simulink model "ACStesbed1"  (R2013b)
settings: Solver=ode45  StartTime=0.0  StopTime=10000  FixedStep=0.01  RelTol=1e-3
StartFcn:
  | InitializeModel
undefined symbols (not defined in the file or in its folder): DiscIntNeverNeededParam, e0_0, e1_0, e2_0, e3_0, magnitude, OrbData, params
libraries: aerolibutil x29, vrlib x26, satellite_control_lib x17, aerolibtransform2 x5, dspmtrx3 x5, aerolib6dofsys x4, dspinverses x3, simulink x3, aerolib6dof2 x1
(part 1 of 2)
settings Model: Creator=DNikolaev  LastModifiedBy=DNikolaev

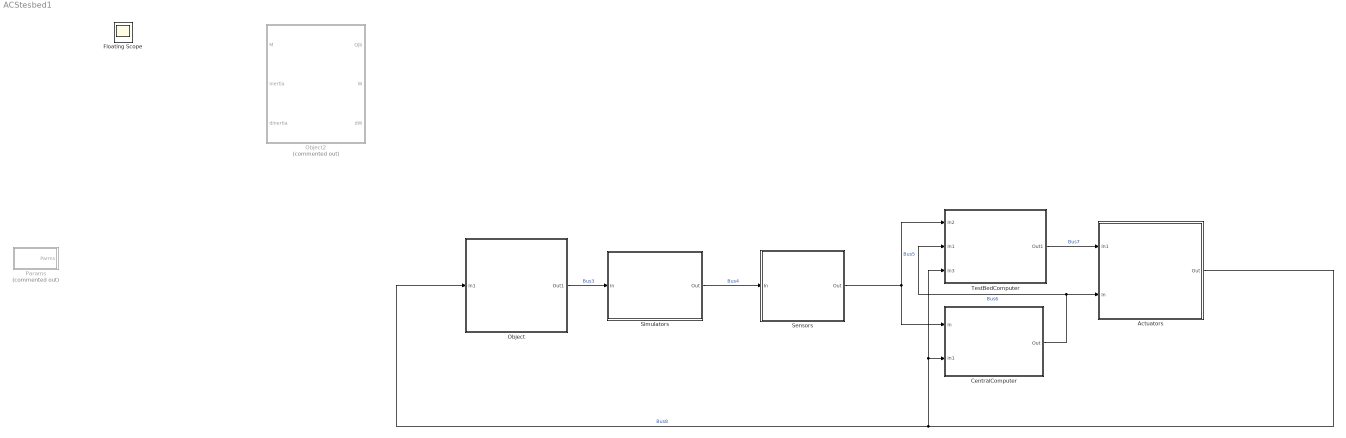
== system ACStesbed1 ==
  Actuators : Subsystem
      mask Display: image('ReactionWheel.gif','center','off')
  CentralComputer : Subsystem
      mask Display: image('cc.jpg')
  Object : Subsystem
  Object2 : Subsystem  Commented=on
      mask Display: image('abtestbed.jpg')
  Params : Subsystem  Commented=on
  Sensors : Subsystem
      mask Display: image('gyro.jpg')
  Simulators : Subsystem
      mask Display: image('space.jpg')
  TestBedComputer : Subsystem
      mask Display: image('computer.jpg')
  Floating Scope : Scope
      settings: Floating=on  SaveName=ScopeData2
  wires:
  Simulators/1(Out) -> Sensors/1(In)  "Bus4"
  Sensors/1(Out) -> CentralComputer/1(In), TestBedComputer/1(In2)  "Bus5"
  Actuators/1(Out) -> Object/1(In1), TestBedComputer/3(In3), CentralComputer/2(In1)  "Bus8"
  CentralComputer/1(Out) -> TestBedComputer/2(In1), Actuators/2(In)  "Bus6"
  TestBedComputer/1(Out1) -> Actuators/1(In1)  "Bus7"
  Object/1(Out1) -> Simulators/1(In)  "Bus3"

== system ACStesbed1/Actuators ==
  In1 : Inport
  In : Inport  Port=2
  Bus Creator : BusCreator  Inputs=7
  Bus Selector1 : BusSelector  OutputSignals=ddeltaD
  Bus Selector4 : BusSelector  OutputSignals=Urw
  Constant : Constant  Value=zeros(3,1)
  Constant1 : Constant  Value=zeros(3,1)
  Gain : Gain
  Gain1 : Gain
  RWmodel : Subsystem
  Subsystem : Subsystem
  Out : Outport
  wires:
  In/1 -> Bus Selector4/1
  Bus Creator/1 -> Out/1
  RWmodel/2(dh) -> Gain/1, Bus Creator/2  "dh"
  Constant/1 -> Bus Creator/5  "L"
  Constant1/1 -> Bus Creator/6  "L_mes"
  Subsystem/1(deltaD) -> Bus Creator/7  "deltaD"
  Bus Selector4/1 -> RWmodel/1(Urw)  "<Urw>"
  RWmodel/1(h) -> Bus Creator/1, Gain1/1  "h"
  Gain/1 -> Bus Creator/4  "dh_mes"
  Gain1/1 -> Bus Creator/3  "h_mes"
  In1/1 -> Bus Selector1/1
  Bus Selector1/1 -> Subsystem/1(ddeltaD)  "<ddeltaD>"

== system ACStesbed1/CentralComputer ==
  In : Inport
  In1 : Inport  Port=2
  Bus Creator : BusCreator  Inputs=5
  Bus Selector : BusSelector  OutputSignals=W_mes,rj2000_mes,vj2000_mes,Qjb_starmes,B_mes,Rsun_mes
  Bus Selector1 : BusSelector  OutputSignals=h_mes
  Constant : Constant  Value=params.g
  Constant3 : Constant  Value=params.Mass
  ModelOfObject : Subsystem
  Quaternion Rotation : aerolibutil/Quaternion Rotation
  SPAttitude : Subsystem
  SatAttitude : Subsystem
  Out : Outport
  wires:
  In/1 -> Bus Selector/1
  Bus Creator/1 -> Out/1
  Bus Selector/1 -> ModelOfObject/1(W), SatAttitude/1(W_mes)  "<W_mes>"
  Bus Selector/2 -> SatAttitude/2(rj2000_mes)  "<rj2000_mes>"
  Bus Selector/3 -> SatAttitude/3(vj2000_mes)  "<vj2000_mes>"
  Bus Selector/4 -> SatAttitude/4(Qjb_starmes)  "<Qjb_starmes>"
  Bus Selector/5 -> SatAttitude/5(B_mes)  "<B_mes>"
  Bus Selector/6 -> SatAttitude/6(Rsun_mes)  "<Rsun_mes>"
  ModelOfObject/1(J_est) -> Bus Creator/1, SatAttitude/7(J_mes)  "J_mes"
  SatAttitude/1(Urw) -> Bus Creator/2  "Urw"
  ModelOfObject/2(dJ_est) -> SatAttitude/8(dJ_mes)
  ModelOfObject/3(h_mes) -> SatAttitude/9(h_mes)
  In1/1 -> Bus Selector1/1
  Bus Selector1/1 -> ModelOfObject/3(h)  "<h_mes>"
  Constant3/1 -> ModelOfObject/2(Mass)
  Constant/1 -> Quaternion Rotation/2  "g"
  SatAttitude/3(Qjb_mes) -> Bus Creator/4  "Qjb_mes"
  Quaternion Rotation/1 -> ModelOfObject/4(g_b)  "g_b"
  SatAttitude/2(dW) -> Bus Creator/3  "dW"
  SatAttitude/4(Qob_mes) -> Bus Creator/5, Quaternion Rotation/1  "Qob_mes"

== system ACStesbed1/Object ==
  In1 : Inport
  Bus Creator{,1..3} (4 alike) : BusCreator  Inputs=2
  Bus Selector : BusSelector  OutputSignals=Bus8.deltaD
  Bus Selector1 : BusSelector  OutputSignals=vj2000,j2000
  From Workspace : FromWorkspace  VariableName=InData  OutDataTypeStr=Bus: BusObject  SampleTime=0  OutputAfterFinalValue=Holding final value
  Inertia : Subsystem
  OrbitalBasis : Subsystem
  TestBedDynamics : Subsystem
      mask Display: image('abtestbed.jpg')
  Torques : Subsystem
  Out1 : Outport
  wires:
  TestBedDynamics/1(Qjb) -> Bus Creator/1  "Qjb"
  TestBedDynamics/2(Omega) -> Bus Creator/2  "W"
  Inertia/1(Inertia) -> TestBedDynamics/2(Inertia)
  Torques/1(T) -> TestBedDynamics/1(M)
  From Workspace/1 -> Bus Selector1/1, Bus Creator1/2  "Bus1"
  Bus Selector1/1 -> OrbitalBasis/1(vj2000)  "<vj2000>"
  Bus Selector1/2 -> OrbitalBasis/2(rj2000)  "<j2000>"
  Bus Creator/1 -> Bus Creator2/1, Bus Creator1/1
  Bus Creator1/1 -> Out1/1  "Bus3"
  Bus Creator2/1 -> Torques/1(InData)
  Inertia/2(dInertia) -> TestBedDynamics/3(dInertia)
  In1/1 -> Bus Creator3/1
  OrbitalBasis/1(Qjo) -> Bus Creator3/2
  Bus Creator3/1 -> Bus Selector/1, Bus Creator2/2
  Bus Selector/1 -> Inertia/1(deltaD)  "<deltaD>"

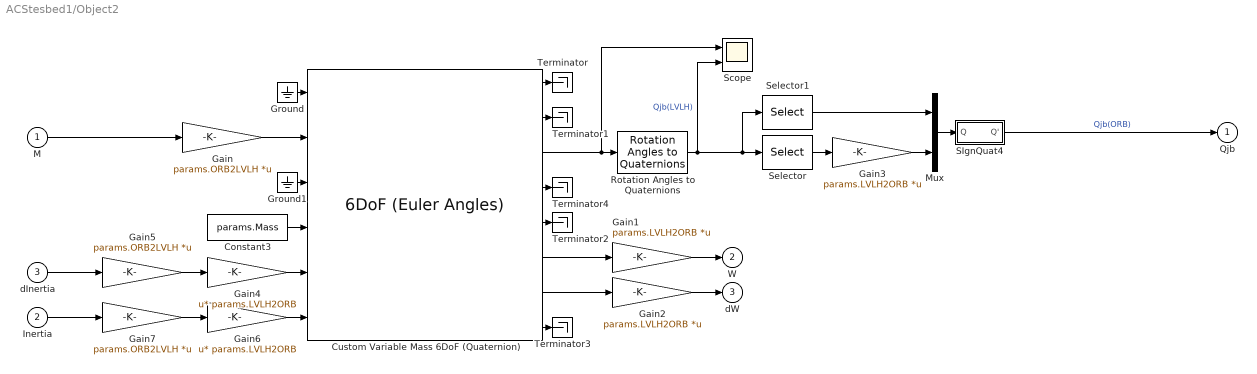
== system ACStesbed1/Object2 ==
  M : Inport
  Inertia : Inport  Port=2
  dInertia : Inport  Port=3
  Constant3 : Constant  Value=params.Mass
  Custom Variable Mass 6DoF (Quaternion) : aerolib6dof2/6DoF (Euler Angles)  units=Metric (MKS)  mtype=Custom Variable  rep=Quaternion  xme_0=[0 0 0]  Vm_0=[0 0 0]  eul_0=[params.roll,params.pitch,params.yaw]  pm_0=params.ORB2LVLH*params.W_b  mass_0=1.0  mass_e=0  mass_f=0  inertia=eye(3)  inertia_e=eye(3)  inertia_f=eye(3)  k_quat=1.0
  Gain : Gain  Gain=params.ORB2LVLH  Multiplication=Matrix(K*u) (u vector)
  Gain1 : Gain  Gain=params.LVLH2ORB  Multiplication=Matrix(K*u) (u vector)
  Gain2 : Gain  Gain=params.LVLH2ORB  Multiplication=Matrix(K*u) (u vector)
  Gain3 : Gain  Gain=params.LVLH2ORB  Multiplication=Matrix(K*u) (u vector)
  Gain4 : Gain  Gain=params.LVLH2ORB  Multiplication=Matrix(u*K)
  Gain5 : Gain  Gain=params.ORB2LVLH  Multiplication=Matrix(K*u)
  Gain6 : Gain  Gain=params.LVLH2ORB  Multiplication=Matrix(u*K)
  Gain7 : Gain  Gain=params.ORB2LVLH  Multiplication=Matrix(K*u)
  Ground : Ground
  Ground1 : Ground
  Mux : Mux  Inputs=2
  Rotation Angles to Quaternions : aerolibtransform2/Rotation Angles to Quaternions  rotationOrder=XYZ
  SIgnQuat4 : Subsystem
  Scope : Scope  NumInputPorts=2
      settings: ShowLegends=on  YMin=-3.25~-0.9  YMax=1.75~1  SaveName=ScopeData4
  Selector : Selector  InputPortWidth=4  IndexOptions=Index vector (dialog)  Indices=[2 3 4]  OutputSizes=1
  Selector1 : Selector  InputPortWidth=4  IndexOptions=Index vector (dialog)  Indices=1  OutputSizes=1
  Terminator{,1..4} (5 alike) : Terminator
  Qjb : Outport
  W : Outport  Port=2
  dW : Outport  Port=3
  wires:
  SIgnQuat4/1(Q') -> Qjb/1  "Qjb(ORB)"
  Mux/1 -> SIgnQuat4/1(Q)
  Constant3/1 -> Custom Variable Mass 6DoF (Quaternion)/4
  Gain6/1 -> Custom Variable Mass 6DoF (Quaternion)/6
  Gain7/1 -> Gain6/1
  Gain4/1 -> Custom Variable Mass 6DoF (Quaternion)/5
  Gain5/1 -> Gain4/1
  Gain3/1 -> Mux/2
  Selector1/1 -> Mux/1
  Selector/1 -> Gain3/1
  Inertia/1 -> Gain7/1
  Custom Variable Mass 6DoF (Quaternion)/3 -> Rotation Angles to Quaternions/1, Scope/1
  Gain2/1 -> dW/1
  Gain1/1 -> W/1
  Gain/1 -> Custom Variable Mass 6DoF (Quaternion)/2
  Custom Variable Mass 6DoF (Quaternion)/4 -> Terminator4/1
  dInertia/1 -> Gain5/1
  M/1 -> Gain/1
  Rotation Angles to Quaternions/1 -> Selector/1, Selector1/1, Scope/2  "Qjb(LVLH)"
  Custom Variable Mass 6DoF (Quaternion)/8 -> Terminator3/1
  Ground/1 -> Custom Variable Mass 6DoF (Quaternion)/1
  Custom Variable Mass 6DoF (Quaternion)/5 -> Terminator2/1
  Custom Variable Mass 6DoF (Quaternion)/1 -> Terminator/1
  Custom Variable Mass 6DoF (Quaternion)/7 -> Gain2/1
  Custom Variable Mass 6DoF (Quaternion)/6 -> Gain1/1
  Ground1/1 -> Custom Variable Mass 6DoF (Quaternion)/3
  Custom Variable Mass 6DoF (Quaternion)/2 -> Terminator1/1

== system ACStesbed1/Params ==
  Bus Creator : BusCreator  Inputs=6
  Constant : Constant  Value=params.invJ_b
  Constant1 : Constant  Value=params.J_b
  Constant2 : Constant  Value=params.Nob
  Constant3 : Constant  Value=params.Mass
  Constant5 : Constant  Value=params.W_b
  Parms : Outport
  wires:
  Bus Creator/1 -> Parms/1
  Constant5/1 -> Bus Creator/5  "W_b_0"
  Constant2/1 -> Bus Creator/4  "Nob_0"
  Constant1/1 -> Bus Creator/2  "Inertia_0"
  Constant/1 -> Bus Creator/1  "invInertia_0"
  Constant3/1 -> Bus Creator/3  "Mass"

== system ACStesbed1/Sensors ==
  In : Inport
  Bus Creator : BusCreator  Inputs=6
  Bus Selector4 : BusSelector  OutputSignals=j2000,vj2000,W,B,Qjb,Rsun
  MagnSensor : Subsystem
  PositionSensor : Subsystem
  RateSensor : Subsystem
      mask Display: text(0.5,0.5,'\omega=(I_3+S)\omega^{true}+\beta^{true}+\eta_\nu','hor','center','texmode','on')
  SIgnQuat : Subsystem
  Scope : Scope  NumInputPorts=2
      settings: ShowLegends=on  YMin=-0.025~-0.025  YMax=0.03~0.03
  StarSensor : Subsystem
  SunSensor : Subsystem
  Out : Outport
  wires:
  Bus Creator/1 -> Out/1
  In/1 -> Bus Selector4/1
  Bus Selector4/3 -> Scope/2, RateSensor/1(W)  "<W>"
  Bus Selector4/4 -> MagnSensor/1(B)  "<B>"
  Bus Selector4/1 -> SunSensor/1(j2000), PositionSensor/1(rj2000)  "<j2000>"
  Bus Selector4/2 -> PositionSensor/2(vj2000)  "<vj2000>"
  Bus Selector4/5 -> SunSensor/2(Qjb), StarSensor/1(Qjb)  "<Qjb>"
  Bus Selector4/6 -> SunSensor/3(Rsun)  "<Rsun>"
  StarSensor/1(Qjb_mes) -> SIgnQuat/1(Q)
  SunSensor/1(Rsun_mes) -> Bus Creator/6  "Rsun_mes"
  MagnSensor/1(B_mes) -> Bus Creator/4  "B_mes"
  RateSensor/1(W_mes) -> Scope/1, Bus Creator/3  "W_mes"
  PositionSensor/2(vj2000_mes) -> Bus Creator/2  "vj2000_mes"
  PositionSensor/1(rj2000_mes) -> Bus Creator/1  "rj2000_mes"
  SIgnQuat/1(Q') -> Bus Creator/5  "Qjb_starmes"

== system ACStesbed1/Simulators ==
  In : Inport
  Bus Creator : BusCreator  Inputs=7
  Bus Selector1 : BusSelector  OutputSignals=signal1.W,signal1.Qjb
  Bus Selector4 : BusSelector  OutputSignals=Bus1.vj2000,Bus1.j2000,Bus1.rsun
  MagnSim : Subsystem
  StarSim : Subsystem
  SunSim : Subsystem
  Out : Outport
  wires:
  Bus Selector4/1 -> Bus Creator/1  "<vj2000>"
  In/1 -> Bus Selector1/1, Bus Selector4/1
  Bus Selector4/2 -> MagnSim/1(j2000), Bus Creator/2  "<j2000>"
  StarSim/1(Out) -> Bus Creator/3  "Stars"
  MagnSim/1(B) -> Bus Creator/4  "B"
  SunSim/1(Rsun_out) -> Bus Creator/5  "Rsun"
  Bus Creator/1 -> Out/1
  Bus Selector4/3 -> SunSim/1(Rsun)  "<rsun>"
  Bus Selector1/1 -> Bus Creator/6  "<W>"
  Bus Selector1/2 -> StarSim/1(In), Bus Creator/7  "<Qjb>"

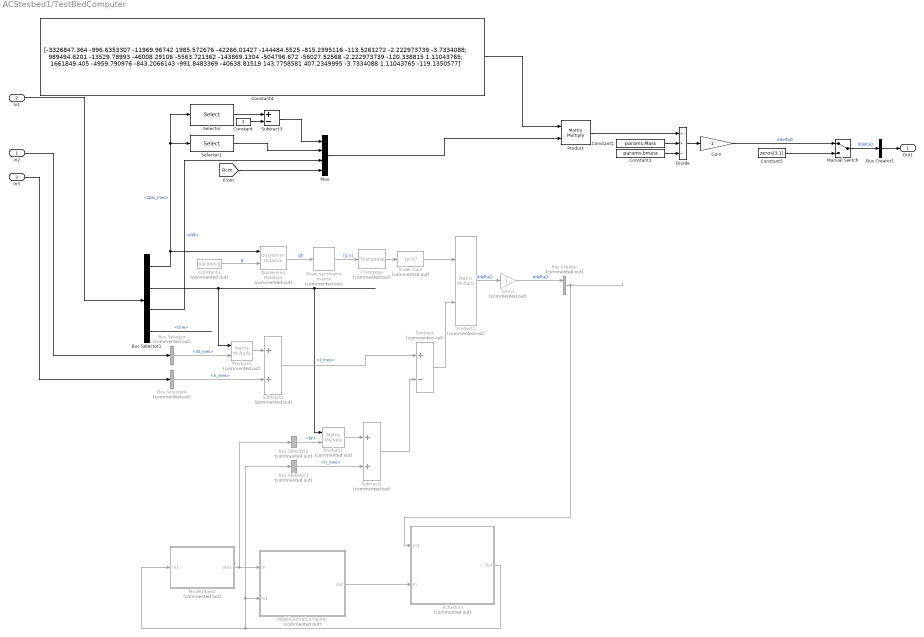
== system ACStesbed1/TestBedComputer ==
  In2 : Inport
  In1 : Inport  Port=2
  In3 : Inport  Port=3
  Actuators : Subsystem  Commented=on
      mask Display: image('ReactionWheel.gif','center','off')
  Bus Creator : BusCreator  Commented=on  Inputs=2
  Bus Creator1 : BusCreator  Inputs=1
  Bus Selector : BusSelector  Commented=on  OutputSignals=W_mes
  Bus Selector1 : BusSelector  OutputSignals=Qob_mes,J_mes,dW,Urw
  Bus Selector2 : BusSelector  Commented=on  OutputSignals=signal1.W
  Bus Selector3 : BusSelector  Commented=on  OutputSignals=h_mes
  Bus Selector4 : BusSelector  Commented=on  OutputSignals=h_mes
  Constant : Constant
  Constant1 : Constant  Value=params.Mass
  Constant2 : Constant  Commented=on  Value=params.g
  Constant3 : Constant  Value=params.bmass
  Constant4 : Constant  Value=|
      | [-3326847.364	-996.6353307	-11969.96742	1985.572676	-42266.01427	-144484.5525	-815.2395116	-113.5261272	-2.222973739	-3.7334088;
      | 989494.6201	-13529.78993	-46008.29106	-5563.721362	-143869.1304	-504796.672	-56027.52568	-2.222973739	-120.338815	1.11043765;
      | 1661849.405	-4959.790976	-843.2066143	-991.8483369	-40638.81519	143.7758581	407.2349995	-3.7334088	1.11043765	-119.1350577]
  Constant5 : Constant  Value=zeros(3,1)
  Divide : Product  Inputs=**/
  Gain : Gain  Gain=-1
  Gain1 : Gain  Commented=on  Gain=-1
  Manual Switch : ManualSwitch
  ModelCentralComputer : Subsystem  Commented=on
      mask Display: image('cc.jpg')
  ModelObject : Subsystem  Commented=on
  Mux : Mux
  Product : Product  Multiplication=Matrix(*)
  Product1 : Product  Commented=on  Multiplication=Matrix(*)
  Product2 : Product  Commented=on  Multiplication=Matrix(*)
  Product3 : Product  Commented=on  Multiplication=Matrix(*)
  Quaternion Rotation : aerolibutil/Quaternion Rotation  Commented=on
  Selector : Selector  InputPortWidth=4  IndexOptions=Index vector (dialog)  Indices=[1 ]  OutputSizes=1
  Selector1 : Selector  InputPortWidth=4  IndexOptions=Index vector (dialog)  Indices=[2 3 4 ]  OutputSizes=1
  Skew-symmetric matrix : satellite_control_lib/Skew-symmetric matrix  Commented=on
  Slider Gain : simulink/Math Operations/Slider Gain  Commented=on  low=0  gain=1e-07  high=1
  Subtract : Sum  Commented=on  Inputs=+-
  Subtract1 : Sum  Commented=on
  Subtract2 : Sum  Commented=on
  Subtract3 : Sum  Inputs=+-
  Transpose : dspmtrx3/Transpose  Commented=on  Hermitian=off  overflowFlag=off
  Out1 : Outport
  wires:
  In2/1 -> Bus Selector/1
  Bus Creator/1 -> Actuators/1(In1)
  ? -> Bus Creator/2  "blabla"
  Product1/1 -> Gain1/1  "ddeltaD"
  In1/1 -> Bus Selector1/1
  Constant2/1 -> Quaternion Rotation/2  "g"
  Bus Selector1/1 -> Selector1/1, Selector/1, Quaternion Rotation/1  "<Qob_mes>"
  Quaternion Rotation/1 -> Skew-symmetric matrix/1  "gb"
  Skew-symmetric matrix/1 -> Transpose/1  "[g x]"
  Bus Selector1/2 -> Product2/1, Product3/1  "<J_mes>"
  Transpose/1 -> Slider Gain/1
  Gain1/1 -> Bus Creator/1  "ddeltaD"
  ModelObject/1(Out1) -> Bus Selector2/1, ModelCentralComputer/1(In)
  ModelCentralComputer/1(Out) -> Actuators/2(In)
  Actuators/1(Out) -> Bus Selector3/1, ModelCentralComputer/2(In1), ModelObject/1(In1)
  Bus Selector1/3 -> Mux/3  "<dW>"
  Bus Selector/1 -> Product3/2  "<W_mes>"
  Bus Selector2/1 -> Product2/2  "<W>"
  Subtract/1 -> Product1/2
  Bus Selector1/4 -> ?  "<Urw>"
  Bus Selector3/1 -> Subtract1/2  "<h_mes>"
  Product2/1 -> Subtract1/1
  Subtract1/1 -> Subtract/2
  In3/1 -> Bus Selector4/1
  Product3/1 -> Subtract2/1
  Bus Selector4/1 -> Subtract2/2  "<h_mes>"
  Subtract2/1 -> Subtract/1
  Slider Gain/1 -> Product1/1
  Constant3/1 -> Divide/3
  Constant1/1 -> Divide/2
  Constant4/1 -> Product/1
  Product/1 -> Divide/1
  Divide/1 -> Gain/1
  Gain/1 -> Manual Switch/1  "ddeltaD"
  Selector/1 -> Subtract3/1
  Constant/1 -> Subtract3/2
  Selector1/1 -> Mux/2
  Subtract3/1 -> Mux/1
  [Rcm] -> Mux/4
  Mux/1 -> Product/2
  Bus Creator1/1 -> Out1/1
  Manual Switch/1 -> Bus Creator1/1  "ddeltaD"
  Constant5/1 -> Manual Switch/2

== system ACStesbed1/Actuators/RWmodel ==
  Urw : Inport
  Gain1 : Gain
  Integrator Limited : Integrator  InitialCondition=[0 0 0]  LimitOutput=on  UpperSaturationLimit=100  LowerSaturationLimit=-100
  Rate Transition : RateTransition  OutPortSampleTime=0.01
  Saturation : Saturate
  Scope : Scope  NumInputPorts=2
      settings: ShowLegends=on  YMin=-0.5~-80  YMax=0.5~20  SaveName=ScopeData5
  h : Outport
  dh : Outport  Port=2
  wires:
  Urw/1 -> Rate Transition/1
  Integrator Limited/1 -> Scope/2, h/1  "h"
  Gain1/1 -> Saturation/1  "dh"
  Saturation/1 -> dh/1
  Rate Transition/1 -> Scope/1, Gain1/1, Integrator Limited/1

== system ACStesbed1/Actuators/Subsystem ==
  ddeltaD : Inport
  D scope : Scope  NumInputPorts=2
      settings: ShowLegends=on  YMin=-2.75e+08~-0.1  YMax=1.5e+08~0.1
  Integrator Limited : Integrator  LimitOutput=on  UpperSaturationLimit=0.1  LowerSaturationLimit=-.1
  Rate Transition : RateTransition  OutPortSampleTime=0.01
  deltaD : Outport
  wires:
  Integrator Limited/1 -> D scope/2, deltaD/1  "deltaD"
  ddeltaD/1 -> D scope/1, Rate Transition/1  "ddeltaD"
  Rate Transition/1 -> Integrator Limited/1  "deltaD"

== system ACStesbed1/CentralComputer/ModelOfObject ==
  W : Inport
  Mass : Inport  Port=2
  h : Inport  Port=3
  g_b : Inport  Port=4
  ChangeMe1 : Constant  Value=zeros(3,3)
  ChangeMe2 : Constant  Value=zeros(1,3)
  ChangeMe3 : Constant  Value=params.J_b
  ChangeMe4 : Constant  Value=zeros(3,3)
  Display : Display
  Display1 : Display
  Divide : Product  Inputs=*/
  J_est : Outport
  dJ_est : Outport  Port=2
  h_mes : Outport  Port=3
  R_est : Outport  Port=4
  wires:
  W/1 -> ?
  ? -> Display/1
  ChangeMe1/1 -> dJ_est/1
  ChangeMe2/1 -> h_mes/1
  Divide/1 -> Display1/1
  ? -> Divide/1
  Mass/1 -> Divide/2
  ChangeMe3/1 -> J_est/1
  ChangeMe4/1 -> R_est/1
  h/1 -> ?
  g_b/1 -> ?

== system ACStesbed1/CentralComputer/SPAttitude ==
  In1 : Inport
  Out1 : Outport
  wires:
  In1/1 -> Out1/1

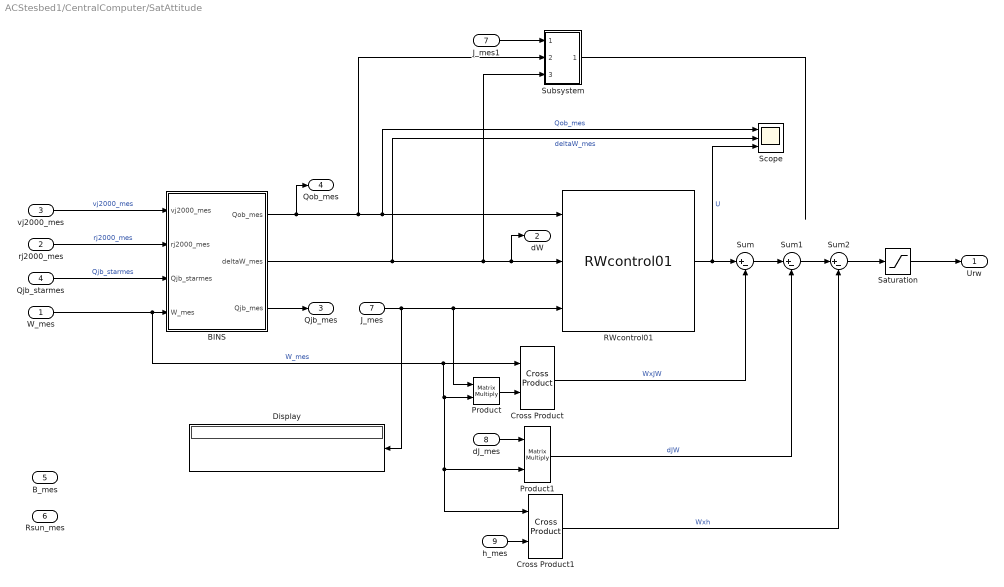
== system ACStesbed1/CentralComputer/SatAttitude ==
  W_mes : Inport
  rj2000_mes : Inport  Port=2
  vj2000_mes : Inport  Port=3
  Qjb_starmes : Inport  Port=4
  B_mes : Inport  Port=5
  Rsun_mes : Inport  Port=6
  J_mes : Inport  Port=7
  dJ_mes : Inport  Port=8
  h_mes : Inport  Port=9
  BINS : Subsystem
  Cross Product : vrlib/Utilities/Cross Product
  Cross Product1 : vrlib/Utilities/Cross Product
  Display : Display
  J_mes1 : InportShadow  Port=7
  Product : Product  Multiplication=Matrix(*)
  Product1 : Product  Multiplication=Matrix(*)
  RWcontrol01 : satellite_control_lib/RWcontrol01  Kq=params.K1acs  Kw=params.K2acs
  Saturation : Saturate
  Scope : Scope  NumInputPorts=3
      settings: ShowLegends=on  YMin=-0.1~-0.00175~-0.2  YMax=1~0.00125~0.9  SaveName=ScopeData7
  Subsystem : Subsystem
  Sum : Sum  Inputs=|+-
  Sum1 : Sum  Inputs=|+-
  Sum2 : Sum  Inputs=|+-
  Urw : Outport
  dW : Outport  Port=2
  Qjb_mes : Outport  Port=3
  Qob_mes : Outport  Port=4
  wires:
  RWcontrol01/1 -> Scope/3, Sum/1  "U"
  vj2000_mes/1 -> BINS/1(vj2000_mes)  "vj2000_mes"
  rj2000_mes/1 -> BINS/2(rj2000_mes)  "rj2000_mes"
  Qjb_starmes/1 -> BINS/3(Qjb_starmes)  "Qjb_starmes"
  W_mes/1 -> Cross Product1/1, Product1/2, Product/2, Cross Product/1, BINS/4(W_mes)  "W_mes"
  J_mes/1 -> Display/1, Product/1, RWcontrol01/3
  BINS/1(Qob_mes) -> Qob_mes/1, Subsystem/2(In2), Scope/1, RWcontrol01/1  "Qob_mes"
  BINS/2(deltaW_mes) -> Scope/2, Subsystem/3(In3), dW/1, RWcontrol01/2  "deltaW_mes"
  J_mes1/1 -> Subsystem/1(In1)
  Subsystem/1(Out1) -> ?
  Saturation/1 -> Urw/1
  Product/1 -> Cross Product/2
  Cross Product/1 -> Sum/2  "WxJW"
  Product1/1 -> Sum1/2  "dJW"
  Cross Product1/1 -> Sum2/2  "Wxh"
  Sum/1 -> Sum1/1
  Sum1/1 -> Sum2/1
  Sum2/1 -> Saturation/1
  h_mes/1 -> Cross Product1/2
  dJ_mes/1 -> Product1/1
  BINS/3(Qjb_mes) -> Qjb_mes/1

== system ACStesbed1/Object/Inertia ==
  deltaD : Inport
  Add : Sum  Inputs=+|+++
  Constant : Constant  Value=zeros(3,3)
  Constant1 : Constant  Value=params.J_b
  Constant2 : Constant  Value=params.be1
  Constant3 : Constant  Value=params.be2
  Constant4 : Constant  Value=params.be3
  Constant5 : Constant  Value=params.rho1
  Constant6 : Constant  Value=params.rho2
  Constant7 : Constant  Value=params.rho3
  Demux : Demux  Outputs=3
  deltaJ1 : Subsystem
  deltaJ2 : Subsystem
  deltaJ3 : Subsystem
  Inertia : Outport
  dInertia : Outport  Port=2
  wires:
  Constant/1 -> dInertia/1
  Constant1/1 -> Add/1  "J0"
  deltaD/1 -> Demux/1
  deltaJ1/1(deltaJ) -> Add/2  "deltaJ1"
  deltaJ2/1(deltaJ) -> Add/3  "deltaJ2"
  deltaJ3/1(deltaJ) -> Add/4  "deltaJ3"
  Add/1 -> Inertia/1  "J0+sum(deltaJ)"
  Demux/1 -> deltaJ1/1(d)
  Demux/2 -> deltaJ2/1(d)
  Demux/3 -> deltaJ3/1(d)
  Constant4/1 -> deltaJ3/2(e)
  Constant3/1 -> deltaJ2/2(e)
  Constant2/1 -> deltaJ1/2(e)
  Constant7/1 -> deltaJ3/3(rho)
  Constant6/1 -> deltaJ2/3(rho)
  Constant5/1 -> deltaJ1/3(rho)

== system ACStesbed1/Object/OrbitalBasis ==
  vj2000 : Inport
  rj2000 : Inport  Port=2
  Cross Product : vrlib/Utilities/Cross Product
  Cross Product1 : vrlib/Utilities/Cross Product
  Direction Cosine Matrix to Quaternions : aerolibtransform2/Direction Cosine Matrix  to Quaternions
  Matrix Concatenate : Concatenate  NumInputs=3  Mode=Multidimensional array  ConcatenateDimension=2
  Normalize Vector : vrlib/Utilities/Normalize Vector  maxzero=0.00001
  Normalize Vector1 : vrlib/Utilities/Normalize Vector  maxzero=0.00001
  Quaternion Conjugate : aerolibutil/Quaternion Conjugate
  Qjo : Outport
  wires:
  Cross Product1/1 -> Matrix Concatenate/1  "iorb"
  Normalize Vector/1 -> Matrix Concatenate/2, Cross Product1/1  "jorb"
  Matrix Concatenate/1 -> Direction Cosine Matrix to Quaternions/1  "DCMjo"
  rj2000/1 -> Normalize Vector/1, Cross Product/2
  vj2000/1 -> Cross Product/1
  Direction Cosine Matrix to Quaternions/1 -> Quaternion Conjugate/1  "Qjo(in J frame)"
  Normalize Vector1/1 -> Matrix Concatenate/3, Cross Product1/2  "korb"
  Cross Product/1 -> Normalize Vector1/1
  Quaternion Conjugate/1 -> Qjo/1  "Qjo"

== system ACStesbed1/Object/TestBedDynamics ==
  M : Inport
  Inertia : Inport  Port=2
  dInertia : Inport  Port=3
  Constant : Constant  Value=params.W_b
  Constant1 : Constant  Value=params.Qjb
  Cross Product : vrlib/Utilities/Cross Product
  Divide : Product  Inputs=/*  Multiplication=Matrix(*)
  Inertia1 : InportShadow  Port=2
  Integrator : Integrator  InitialConditionSource=external
  Product : Product  Multiplication=Matrix(*)
  Product1 : Product  Multiplication=Matrix(*)
  Scope : Scope  NumInputPorts=3
      settings: ShowLegends=on  YMin=-0.005~-0.45~-5  YMax=0.0045~0.2~5  SaveName=ScopeData8
  Sum : Sum  Inputs=+--
  quatint : Subsystem
  Qjb : Outport
  Omega : Outport  Port=2
  wires:
  Sum/1 -> Divide/2
  Inertia1/1 -> Divide/1
  Divide/1 -> Scope/3, Integrator/1  "dOmega"
  Constant/1 -> Integrator/2
  Product/1 -> Sum/2  "dI*Omega"
  dInertia/1 -> Product/1
  Constant1/1 -> quatint/2(q_init)
  quatint/1(q) -> Qjb/1  "Qjb"
  Inertia/1 -> Product1/1
  Product1/1 -> Cross Product/2
  Cross Product/1 -> Sum/3  "Omega x I*Omega"
  Integrator/1 -> Scope/1, quatint/1(p q r), Cross Product/1, Product/2, Product1/2, Omega/1  "W"
  M/1 -> Scope/2, Sum/1  "M"

== system ACStesbed1/Object/Torques ==
  InData : Inport
  Add1 : Sum  Inputs=4
  Bus Selector : BusSelector  OutputSignals=signal2.Bus8.dh,signal1.W,signal2.Bus8.h,signal2.Qjo,signal1.Qjb,signal2.Bus8.deltaD,signal2.Bus8.L
  Calc Qob : Subsystem
  ChangeMe : Constant  Value=params.Rcm
  ChangeMe1 : Constant  Value=[0 0 0]
  Saturation : Saturate  UpperLimit=1  LowerLimit=-1
  SignQuat : Subsystem
  Tgrav : Subsystem
  Tm : Subsystem
  Torques scope : Scope  NumInputPorts=2
      settings: ShowLegends=on  YMin=-0.55~-0.025  YMax=0.1~0.4  SaveName=ScopeData3
  Tothers : Subsystem
  Trw : Subsystem
  T : Outport
  wires:
  InData/1 -> Bus Selector/1
  Bus Selector/7 -> Tm/1(L)  "<L>"
  Bus Selector/6 -> Tgrav/3(deltaD)  "<deltaD>"
  Add1/1 -> T/1
  Bus Selector/1 -> Trw/1(dh)  "<dh>"
  Bus Selector/2 -> Trw/2(W)  "<W>"
  Bus Selector/3 -> Trw/3(h)  "<h>"
  Trw/1(Trw) -> Saturation/1  "Trw_"
  Tgrav/1(Tg) -> Torques scope/2, Add1/2  "Tg"
  Tm/1(Tm) -> ?  "Tm"
  Tothers/1(Tothers) -> ?  "Tothers"
  ChangeMe1/1 -> Tothers/1(Something), Tm/3(Ldisturb), Tm/2(B)
  Saturation/1 -> Torques scope/1, Add1/1  "Trw"
  ChangeMe/1 -> Tgrav/2(Rcm0)
  Calc Qob/1(Qob) -> SignQuat/1(Q)
  Bus Selector/5 -> Calc Qob/2(Qjb)  "<Qjb>"
  Bus Selector/4 -> Calc Qob/1(Qjo)  "<Qjo>"
  SignQuat/1(Q') -> Tgrav/1(Qob)

== system ACStesbed1/Object2/SIgnQuat4 ==
  Q : Inport
  Constant : Constant
  Constant1 : Constant  Value=-1
  Product : Product
  Selector2 : Selector  InputPortWidth=4  IndexOptions=Index vector (dialog)  Indices=[1]  OutputSizes=1
  Switch : Switch
  Q' : Outport
  wires:
  Constant1/1 -> Switch/3
  Constant/1 -> Switch/1
  Selector2/1 -> Switch/2
  Switch/1 -> Product/1
  Product/1 -> Q'/1
  Q/1 -> Selector2/1, Product/2

== system ACStesbed1/Sensors/MagnSensor ==
  B : Inport
  Noise : Constant  Value=[0 0 0]
  Sum : Sum  Inputs=|++
  Zero-Order Hold : ZeroOrderHold  SampleTime=0.1
  B_mes : Outport
  wires:
  B/1 -> Sum/1
  Noise/1 -> Sum/2
  Sum/1 -> Zero-Order Hold/1
  Zero-Order Hold/1 -> B_mes/1

== system ACStesbed1/Sensors/PositionSensor ==
  rj2000 : Inport
  vj2000 : Inport  Port=2
  Noise : Constant  Value=[0 0 0]
  Noise1 : Constant  Value=[0 0 0]
  Sum : Sum  Inputs=|++
  Sum1 : Sum  Inputs=|++
  Zero-Order Hold : ZeroOrderHold  SampleTime=0.1
  Zero-Order Hold1 : ZeroOrderHold  SampleTime=0.1
  rj2000_mes : Outport
  vj2000_mes : Outport  Port=2
  wires:
  rj2000/1 -> Sum/1
  Noise/1 -> Sum/2
  Sum/1 -> Zero-Order Hold/1
  Zero-Order Hold/1 -> rj2000_mes/1
  vj2000/1 -> Sum1/1
  Noise1/1 -> Sum1/2
  Sum1/1 -> Zero-Order Hold1/1
  Zero-Order Hold1/1 -> vj2000_mes/1

== system ACStesbed1/Sensors/RateSensor ==
  W : Inport
  Add : Sum
  Band-Limited White Noise : simulink/Sources/Band-Limited White Noise  Cov=params.VarRSB/0.1  Ts=0.1  seed=[23341]
  Band-Limited White Noise1 : simulink/Sources/Band-Limited White Noise  Cov=params.VarRSN/0.1  Ts=0.1  seed=[23341]
  Constant : Constant  Value=params.RSSE
  I3 : dspmtrx3/Constant Diagonal Matrix  q=ones(1,3)  frame=off  dataType=Inherit from 'Constant(s) along diagonal'  isSigned=on  wordLen=16  udDataType=sfix(16)  fracBitsMode=Best precision  numFracBits=15
  Integrator : Integrator
  Product : Product  Multiplication=Matrix(*)
  Sum : Sum  Inputs=|++
  Sum1 : Sum  Inputs=|++
  Zero-Order Hold : ZeroOrderHold  SampleTime=0.1
  W_mes : Outport
  wires:
  W/1 -> Product/2
  Sum/1 -> Zero-Order Hold/1
  Zero-Order Hold/1 -> W_mes/1
  Sum1/1 -> Sum/1
  I3/1 -> Add/1
  Constant/1 -> Add/2
  Add/1 -> Product/1
  Product/1 -> Sum1/1
  Band-Limited White Noise1/1 -> Sum/2  "noise"
  Integrator/1 -> Sum1/2  "Bias"
  Band-Limited White Noise/1 -> Integrator/1  "dBias"

== system ACStesbed1/Sensors/SIgnQuat ==
  Q : Inport
  Product : Product
  Selector2 : Selector  InputPortWidth=4  IndexOptions=Index vector (dialog)  Indices=[1]  OutputSizes=1
  Sign : Signum
  Q' : Outport
  wires:
  Q/1 -> Product/2, Selector2/1
  Product/1 -> Q'/1
  Sign/1 -> Product/1
  Selector2/1 -> Sign/1

== system ACStesbed1/Sensors/StarSensor ==
  Qjb : Inport
  Noise : Constant  Value=[0 0 0 0]
  Sum : Sum  Inputs=|++
  Zero-Order Hold : ZeroOrderHold  SampleTime=0.1
  Qjb_mes : Outport
  wires:
  Zero-Order Hold/1 -> Qjb_mes/1
  Qjb/1 -> Sum/1
  Noise/1 -> Sum/2
  Sum/1 -> Zero-Order Hold/1

== system ACStesbed1/Sensors/SunSensor ==
  j2000 : Inport
  Qjb : Inport  Port=2
  Rsun : Inport  Port=3
  Gain : Gain  Gain=params.au2km
  Noise : Constant  Value=[0 0 0]
  Normalize Vector : vrlib/Utilities/Normalize Vector  maxzero=0
  Quaternion Rotation : aerolibutil/Quaternion Rotation
  Subtract : Sum  Inputs=|+-
  Sum : Sum  Inputs=|++
  Zero-Order Hold : ZeroOrderHold  SampleTime=0.1
  Rsun_mes : Outport
  wires:
  Rsun/1 -> Gain/1
  Gain/1 -> Subtract/1
  j2000/1 -> Subtract/2
  Subtract/1 -> Quaternion Rotation/2  "rrsun"
  Qjb/1 -> Quaternion Rotation/1
  Quaternion Rotation/1 -> Normalize Vector/1
  Zero-Order Hold/1 -> Rsun_mes/1  "Rsun_mes"
  Normalize Vector/1 -> Sum/1  "rrsuno"
  Noise/1 -> Sum/2
  Sum/1 -> Zero-Order Hold/1

== system ACStesbed1/Simulators/MagnSim ==
  j2000 : Inport
  B : Outport
  wires:
  j2000/1 -> B/1

== system ACStesbed1/Simulators/StarSim ==
  In : Inport
  Out : Outport
  wires:
  In/1 -> Out/1

== system ACStesbed1/Simulators/SunSim ==
  Rsun : Inport
  Rsun_out : Outport
  wires:
  Rsun/1 -> Rsun_out/1

== system ACStesbed1/TestBedComputer/Actuators ==
  In1 : Inport
  In : Inport  Port=2
  Bus Creator : BusCreator  Inputs=7
  Bus Selector1 : BusSelector  OutputSignals=ddeltaD
  Bus Selector4 : BusSelector  OutputSignals=Urw
  Constant : Constant  Value=zeros(3,1)
  Constant1 : Constant  Value=zeros(3,1)
  Gain : Gain
  Gain1 : Gain
  RWmodel : Subsystem
  Subsystem : Subsystem
  Out : Outport
  wires:
  In/1 -> Bus Selector4/1
  Bus Creator/1 -> Out/1
  RWmodel/2(dh) -> Gain/1, Bus Creator/2  "dh"
  Constant/1 -> Bus Creator/5  "L"
  Constant1/1 -> Bus Creator/6  "L_mes"
  Subsystem/1(deltaD) -> Bus Creator/7  "deltaD"
  Bus Selector4/1 -> RWmodel/1(Urw)  "<Urw>"
  RWmodel/1(h) -> Bus Creator/1, Gain1/1  "h"
  Gain/1 -> Bus Creator/4  "dh_mes"
  Gain1/1 -> Bus Creator/3  "h_mes"
  In1/1 -> Bus Selector1/1
  Bus Selector1/1 -> Subsystem/1(ddeltaD)  "<ddeltaD>"

== system ACStesbed1/TestBedComputer/ModelCentralComputer ==
  In : Inport
  In1 : Inport  Port=2
  Bus Creator : BusCreator  Inputs=5
  Bus Selector : BusSelector  OutputSignals=signal1.W,Bus1.j2000,Bus1.vj2000,signal1.Qjb,Bus1.rsun
  Bus Selector1 : BusSelector  OutputSignals=h_mes
  Constant : Constant  Value=params.g
  Constant3 : Constant  Value=params.Mass
  ModelOfObject : Subsystem
  Quaternion Rotation : aerolibutil/Quaternion Rotation
  SPAttitude : Subsystem
  SatAttitude : Subsystem
  Out : Outport
  wires:
  In/1 -> Bus Selector/1
  Bus Creator/1 -> Out/1
  Bus Selector/1 -> ModelOfObject/1(W), SatAttitude/1(W_mes)  "<W>"
  Bus Selector/2 -> SatAttitude/2(rj2000_mes)  "<j2000>"
  Bus Selector/3 -> SatAttitude/3(vj2000_mes)  "<vj2000>"
  Bus Selector/4 -> SatAttitude/4(Qjb_starmes)  "<Qjb>"
  ? -> SatAttitude/5(B_mes)
  Bus Selector/5 -> SatAttitude/6(Rsun_mes)  "<rsun>"
  ModelOfObject/1(J_est) -> Bus Creator/1, SatAttitude/7(J_mes)  "J_mes"
  SatAttitude/1(Urw) -> Bus Creator/2  "Urw"
  ModelOfObject/2(dJ_est) -> SatAttitude/8(dJ_mes)
  ModelOfObject/3(h_mes) -> SatAttitude/9(h_mes)
  In1/1 -> Bus Selector1/1
  Bus Selector1/1 -> ModelOfObject/3(h)  "<h_mes>"
  Constant3/1 -> ModelOfObject/2(Mass)
  Constant/1 -> Quaternion Rotation/2  "g"
  SatAttitude/3(Qjb_mes) -> Bus Creator/4  "Qjb_mes"
  Quaternion Rotation/1 -> ModelOfObject/4(g_b)  "g_b"
  SatAttitude/2(dW) -> Bus Creator/3  "dW"
  SatAttitude/4(Qob_mes) -> Bus Creator/5, Quaternion Rotation/1  "Qob_mes"

== system ACStesbed1/TestBedComputer/ModelObject ==
  In1 : Inport
  Bus Creator{,1..3} (4 alike) : BusCreator  Inputs=2
  Bus Selector : BusSelector  OutputSignals=signal1.deltaD
  Bus Selector1 : BusSelector  OutputSignals=vj2000,j2000
  From Workspace : FromWorkspace  VariableName=InData  OutDataTypeStr=Bus: BusObject  SampleTime=0  OutputAfterFinalValue=Holding final value
  Inertia : Subsystem
  OrbitalBasis : Subsystem
  TestBedDynamics : Subsystem
      mask Display: image('abtestbed.jpg')
  Torques : Subsystem
  Out1 : Outport
  wires:
  TestBedDynamics/1(Qjb) -> Bus Creator/1  "Qjb"
  TestBedDynamics/2(Omega) -> Bus Creator/2  "W"
  Inertia/1(Inertia) -> TestBedDynamics/2(Inertia)
  Torques/1(T) -> TestBedDynamics/1(M)
  From Workspace/1 -> Bus Selector1/1, Bus Creator1/2  "Bus1"
  Bus Selector1/1 -> OrbitalBasis/1(vj2000)  "<vj2000>"
  Bus Selector1/2 -> OrbitalBasis/2(rj2000)  "<j2000>"
  Bus Creator/1 -> Bus Creator2/1, Bus Creator1/1
  Bus Creator1/1 -> Out1/1  "Bus3"
  Bus Creator2/1 -> Torques/1(InData)
  Inertia/2(dInertia) -> TestBedDynamics/3(dInertia)
  In1/1 -> Bus Creator3/1
  OrbitalBasis/1(Qjo) -> Bus Creator3/2
  Bus Creator3/1 -> Bus Selector/1, Bus Creator2/2
  Bus Selector/1 -> Inertia/1(deltaD)  "<deltaD>"

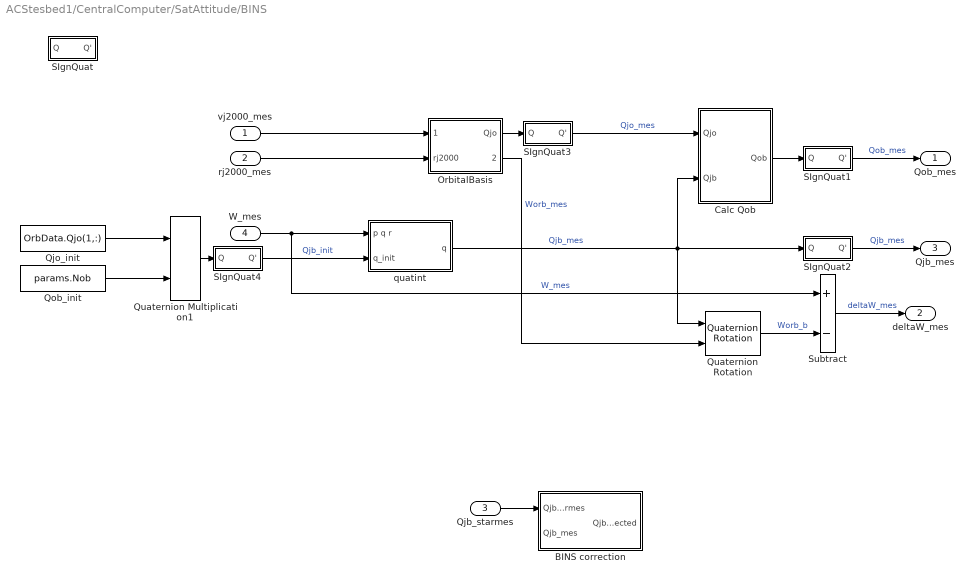
== system ACStesbed1/CentralComputer/SatAttitude/BINS ==
  vj2000_mes : Inport
  rj2000_mes : Inport  Port=2
  Qjb_starmes : Inport  Port=3
  W_mes : Inport  Port=4
  BINS correction : Subsystem
  Calc Qob : Subsystem
  OrbitalBasis : Subsystem
  Qjo_init : Constant  Value=OrbData.Qjo(1,:)
  Qob_init : Constant  Value=params.Nob
  Quaternion Multiplication1 : aerolibutil/Quaternion Multiplication
  Quaternion Rotation : aerolibutil/Quaternion Rotation
  SIgnQuat : Subsystem
  SIgnQuat1 : Subsystem
  SIgnQuat2 : Subsystem
  SIgnQuat3 : Subsystem
  SIgnQuat4 : Subsystem
  Subtract : Sum  Inputs=+-
  quatint : Subsystem
  Qob_mes : Outport
  deltaW_mes : Outport  Port=2
  Qjb_mes : Outport  Port=3
  wires:
  Qjb_starmes/1 -> BINS correction/1(Qjb_starmes)
  quatint/1(q) -> SIgnQuat2/1(Q), Calc Qob/2(Qjb), Quaternion Rotation/1  "Qjb_mes"
  Calc Qob/1(Qob) -> SIgnQuat1/1(Q)
  rj2000_mes/1 -> OrbitalBasis/2(rj2000)
  vj2000_mes/1 -> OrbitalBasis/1(vj2000)
  OrbitalBasis/1(Qjo) -> SIgnQuat3/1(Q)
  OrbitalBasis/2(Worb_j) -> Quaternion Rotation/2  "Worb_mes"
  W_mes/1 -> Subtract/1, quatint/1(p q r)  "W_mes"
  Subtract/1 -> deltaW_mes/1  "deltaW_mes"
  Qjo_init/1 -> Quaternion Multiplication1/1
  Qob_init/1 -> Quaternion Multiplication1/2
  Quaternion Multiplication1/1 -> SIgnQuat4/1(Q)
  Quaternion Rotation/1 -> Subtract/2  "Worb_b"
  SIgnQuat1/1(Q') -> Qob_mes/1  "Qob_mes"
  SIgnQuat2/1(Q') -> Qjb_mes/1  "Qjb_mes"
  SIgnQuat3/1(Q') -> Calc Qob/1(Qjo)  "Qjo_mes"
  SIgnQuat4/1(Q') -> quatint/2(q_init)  "Qjb_init"

== system ACStesbed1/CentralComputer/SatAttitude/Subsystem ==
  In1 : Inport
  In2 : Inport  Port=2
  In3 : Inport  Port=3
  Gain : Gain  Gain=-1
  Product5 : Product  Multiplication=Matrix(*)
  Selector : Selector  InputPortWidth=4  IndexOptions=Index vector (dialog)  Indices=1  OutputSizes=1
  Selector1 : Selector  InputPortWidth=4  IndexOptions=Index vector (dialog)  Indices=[2 3 4]  OutputSizes=1
  Subsystem1 : Subsystem
  a : Constant  Value=-0.9
  Out1 : Outport
  wires:
  Subsystem1/1(Trw) -> Product5/2
  Selector1/1 -> Subsystem1/3(q)
  a/1 -> Subsystem1/1(a)
  Selector/1 -> Subsystem1/2(q0)  "1"
  Product5/1 -> Gain/1
  In2/1 -> Selector1/1, Selector/1
  In3/1 -> Subsystem1/4(w)
  In1/1 -> Product5/1
  Gain/1 -> Out1/1

== system ACStesbed1/Object/Inertia/deltaJ1 ==
  d : Inport
  e : Inport  Port=2
  rho : Inport  Port=3
  Add : Sum  Inputs=3
  Constant : Constant  Value=params.bmass
  Gain : Gain  Gain=-1
  Math Function : Math  Operator=magnitude^2  SaturateOnIntegerOverflow=on
  Product{,4..6} (4 alike) : Product
  Product1 : Product  Multiplication=Matrix(*)
  Product2 : Product  Multiplication=Matrix(*)
  Product3 : Product  Multiplication=Matrix(*)
  Skew-symmetric matrix : satellite_control_lib/Skew-symmetric matrix
  Skew-symmetric matrix1 : satellite_control_lib/Skew-symmetric matrix
  deltaJ : Outport
  wires:
  Constant/1 -> Gain/1
  e/1 -> Skew-symmetric matrix/1
  rho/1 -> Skew-symmetric matrix1/1
  Product/1 -> deltaJ/1  "(-m)(d^2[e x]^2+d[rho x][e x]+d[e x][rho x])"
  Gain/1 -> Product/1
  d/1 -> Math Function/1, Product6/1, Product5/1
  Skew-symmetric matrix/1 -> Product2/2, Product3/1, Product1/1, Product1/2  "[e x]"
  Math Function/1 -> Product4/1
  Product1/1 -> Product4/2
  Skew-symmetric matrix1/1 -> Product3/2, Product2/1  "[rho x]"
  Product3/1 -> Product5/2
  Product2/1 -> Product6/2
  Add/1 -> Product/2
  Product4/1 -> Add/1
  Product5/1 -> Add/2
  Product6/1 -> Add/3

== system ACStesbed1/Object/Inertia/deltaJ2 ==
  d : Inport
  e : Inport  Port=2
  rho : Inport  Port=3
  Add : Sum  Inputs=3
  Constant : Constant  Value=params.bmass
  Gain : Gain  Gain=-1
  Math Function : Math  Operator=magnitude^2  SaturateOnIntegerOverflow=on
  Product{,4..6} (4 alike) : Product
  Product1 : Product  Multiplication=Matrix(*)
  Product2 : Product  Multiplication=Matrix(*)
  Product3 : Product  Multiplication=Matrix(*)
  Skew-symmetric matrix : satellite_control_lib/Skew-symmetric matrix
  Skew-symmetric matrix1 : satellite_control_lib/Skew-symmetric matrix
  deltaJ : Outport
  wires:
  Product6/1 -> Add/3
  Product5/1 -> Add/2
  Product4/1 -> Add/1
  Add/1 -> Product/2
  Product2/1 -> Product6/2
  Product3/1 -> Product5/2
  Skew-symmetric matrix1/1 -> Product2/1, Product3/2  "[rho x]"
  Product1/1 -> Product4/2
  Math Function/1 -> Product4/1
  Skew-symmetric matrix/1 -> Product1/2, Product1/1, Product3/1, Product2/2  "[e x]"
  d/1 -> Product5/1, Product6/1, Math Function/1
  Gain/1 -> Product/1
  Product/1 -> deltaJ/1  "(-m)(d^2[e x]^2+d[rho x][e x]+d[e x][rho x])"
  rho/1 -> Skew-symmetric matrix1/1
  e/1 -> Skew-symmetric matrix/1
  Constant/1 -> Gain/1

== system ACStesbed1/Object/Inertia/deltaJ3 ==
  d : Inport
  e : Inport  Port=2
  rho : Inport  Port=3
  Add : Sum  Inputs=3
  Constant : Constant  Value=params.bmass
  Gain : Gain  Gain=-1
  Math Function : Math  Operator=magnitude^2  SaturateOnIntegerOverflow=on
  Product{,4..6} (4 alike) : Product
  Product1 : Product  Multiplication=Matrix(*)
  Product2 : Product  Multiplication=Matrix(*)
  Product3 : Product  Multiplication=Matrix(*)
  Skew-symmetric matrix : satellite_control_lib/Skew-symmetric matrix
  Skew-symmetric matrix1 : satellite_control_lib/Skew-symmetric matrix
  deltaJ : Outport
  wires:
  Constant/1 -> Gain/1
  e/1 -> Skew-symmetric matrix/1
  rho/1 -> Skew-symmetric matrix1/1
  Product/1 -> deltaJ/1  "(-m)(d^2[e x]^2+d[rho x][e x]+d[e x][rho x])"
  Gain/1 -> Product/1
  d/1 -> Math Function/1, Product6/1, Product5/1
  Skew-symmetric matrix/1 -> Product2/2, Product3/1, Product1/1, Product1/2  "[e x]"
  Math Function/1 -> Product4/1
  Product1/1 -> Product4/2
  Skew-symmetric matrix1/1 -> Product3/2, Product2/1  "[rho x]"
  Product3/1 -> Product5/2
  Product2/1 -> Product6/2
  Add/1 -> Product/2
  Product4/1 -> Add/1
  Product5/1 -> Add/2
  Product6/1 -> Add/3

== system ACStesbed1/Object/TestBedDynamics/quatint ==
  p q r : Inport
  q_init : Inport  Port=2
  q0 q1 q2 q3 : Integrator  InitialConditionSource=external  InitialCondition=[e0_0 e1_0 e2_0 e3_0]
  qdot : aerolib6dofsys/DCM & Euler Angles (Quaternion)/qdot
  q : Outport
  wires:
  q0 q1 q2 q3/1 -> q/1, qdot/2
  q_init/1 -> q0 q1 q2 q3/2
  p q r/1 -> qdot/1
  qdot/1 -> q0 q1 q2 q3/1

== system ACStesbed1/Object/Torques/Calc Qob ==
  Qjo : Inport
  Qjb : Inport  Port=2
  Quaternion Inverse : aerolibutil/Quaternion Inverse
  Quaternion Multiplication : aerolibutil/Quaternion Multiplication
  Qob : Outport
  wires:
  Qjb/1 -> Quaternion Multiplication/2  "Qjb"
  Qjo/1 -> Quaternion Inverse/1  "Qjo"
  Quaternion Inverse/1 -> Quaternion Multiplication/1
  Quaternion Multiplication/1 -> Qob/1

== system ACStesbed1/Object/Torques/SignQuat ==
  Q : Inport
  Product : Product
  Selector2 : Selector  InputPortWidth=4  IndexOptions=Index vector (dialog)  Indices=[1]  OutputSizes=1
  Sign : Signum
  Q' : Outport
  wires:
  Q/1 -> Product/2, Selector2/1
  Product/1 -> Q'/1
  Sign/1 -> Product/1
  Selector2/1 -> Sign/1

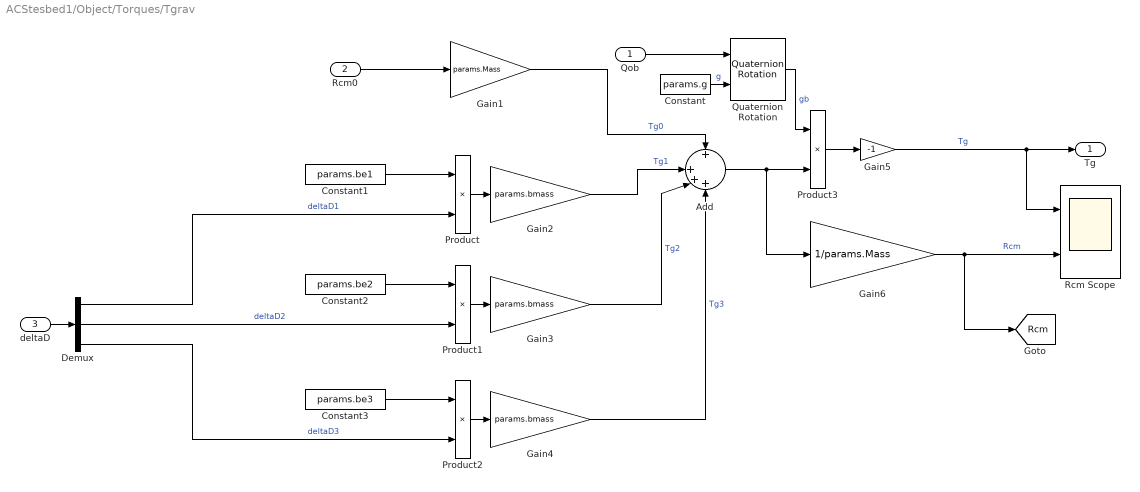
== system ACStesbed1/Object/Torques/Tgrav ==
  Qob : Inport
  Rcm0 : Inport  Port=2
  deltaD : Inport  Port=3
  Add : Sum  Inputs=+|+++
  Constant : Constant  Value=params.g
  Constant1 : Constant  Value=params.be1
  Constant2 : Constant  Value=params.be2
  Constant3 : Constant  Value=params.be3
  Demux : Demux  Outputs=3
  Gain1 : Gain  Gain=params.Mass
  Gain2 : Gain  Gain=params.bmass
  Gain3 : Gain  Gain=params.bmass
  Gain4 : Gain  Gain=params.bmass
  Gain5 : Gain  Gain=-1
  Gain6 : Gain  Gain=1/params.Mass
  Product{,1..3} (4 alike) : Product
  Quaternion Rotation : aerolibutil/Quaternion Rotation
  Rcm Scope : Scope  NumInputPorts=2
      settings: ShowLegends=on  YMin=-0.05~-2e-05  YMax=0.4~0.00014  SaveName=ScopeData6
  Tg : Outport
  tag scope: Rcm=global
  wires:
  Rcm0/1 -> Gain1/1
  Constant/1 -> Quaternion Rotation/2  "g"
  Gain1/1 -> Add/1  "Tg0"
  Constant1/1 -> Product/1
  deltaD/1 -> Demux/1
  Constant2/1 -> Product1/1
  Demux/2 -> Product1/2  "deltaD2"
  Constant3/1 -> Product2/1
  Product/1 -> Gain2/1
  Product1/1 -> Gain3/1
  Product2/1 -> Gain4/1
  Gain2/1 -> Add/2  "Tg1"
  Gain3/1 -> Add/3  "Tg2"
  Gain4/1 -> Add/4  "Tg3"
  Add/1 -> Gain6/1, Product3/2
  Demux/3 -> Product2/2  "deltaD3"
  Demux/1 -> Product/2  "deltaD1"
  Quaternion Rotation/1 -> Product3/1  "gb"
  Product3/1 -> Gain5/1
  Gain5/1 -> Rcm Scope/1, Tg/1  "Tg"
  Qob/1 -> Quaternion Rotation/1
  Gain6/1 -> [Rcm], Rcm Scope/2  "Rcm"

== system ACStesbed1/Object/Torques/Tm ==
  L : Inport
  B : Inport  Port=2
  Ldisturb : Inport  Port=3
  Tm : Outport
  wires:
  L/1 -> Tm/1

== system ACStesbed1/Object/Torques/Tothers ==
  Something : Inport
  Tothers : Outport
  wires:
  Something/1 -> Tothers/1

== system ACStesbed1/Object/Torques/Trw ==
  dh : Inport
  W : Inport  Port=2
  h : Inport  Port=3
  Add : Sum
  Cross Product : vrlib/Utilities/Cross Product
  Gain : Gain  Gain=-1
  Trw : Outport
  wires:
  W/1 -> Cross Product/1
  Gain/1 -> Trw/1  "Trw"
  Cross Product/1 -> Add/2  "Wxh"
  Add/1 -> Gain/1  "(dH+WxH)"
  dh/1 -> Add/1
  h/1 -> Cross Product/2

== system ACStesbed1/TestBedComputer/Actuators/RWmodel ==
  Urw : Inport
  Gain1 : Gain
  Integrator Limited : Integrator  InitialCondition=[0 0 0]  LimitOutput=on  UpperSaturationLimit=100  LowerSaturationLimit=-100
  Rate Transition : RateTransition  OutPortSampleTime=0.01
  Saturation : Saturate
  Scope : Scope  NumInputPorts=2
      settings: ShowLegends=on  YMin=-0.05~-2  YMax=0.03~1  SaveName=ScopeData5
  h : Outport
  dh : Outport  Port=2
  wires:
  Urw/1 -> Rate Transition/1
  Integrator Limited/1 -> Scope/2, h/1  "h"
  Gain1/1 -> Saturation/1  "dh"
  Saturation/1 -> dh/1
  Rate Transition/1 -> Scope/1, Gain1/1, Integrator Limited/1

== system ACStesbed1/TestBedComputer/Actuators/Subsystem ==
  ddeltaD : Inport
  Integrator Limited : Integrator  LimitOutput=on  UpperSaturationLimit=0.4  LowerSaturationLimit=-0.4
  Rate Transition : RateTransition  OutPortSampleTime=0.01
  deltaD scope : Scope  NumInputPorts=2
      settings: ShowLegends=on  YMin=-0.00045~-0.025  YMax=0.0006~0.4  SaveName=ScopeData9
  deltaD : Outport
  wires:
  Integrator Limited/1 -> deltaD scope/2, deltaD/1  "deltaD"
  Rate Transition/1 -> Integrator Limited/1, deltaD scope/1  "ddeltaD"
  ddeltaD/1 -> Rate Transition/1

== system ACStesbed1/TestBedComputer/ModelCentralComputer/ModelOfObject ==
  W : Inport
  Mass : Inport  Port=2
  h : Inport  Port=3
  g_b : Inport  Port=4
  ChangeMe1 : Constant  Value=zeros(3,3)
  ChangeMe2 : Constant  Value=zeros(1,3)
  ChangeMe3 : Constant  Value=params.J_b
  ChangeMe4 : Constant  Value=zeros(3,3)
  Display : Display
  Display1 : Display
  Divide : Product  Inputs=*/
  InertiaIdentification : Subsystem
  J_est : Outport
  dJ_est : Outport  Port=2
  h_mes : Outport  Port=3
  R_est : Outport  Port=4
  wires:
  W/1 -> InertiaIdentification/1(W)
  InertiaIdentification/1(J_est) -> Display/1
  ChangeMe1/1 -> dJ_est/1
  ChangeMe2/1 -> h_mes/1
  Divide/1 -> Display1/1
  InertiaIdentification/2(mr_est) -> Divide/1
  Mass/1 -> Divide/2
  ChangeMe3/1 -> J_est/1
  ChangeMe4/1 -> R_est/1
  h/1 -> InertiaIdentification/2(h)
  g_b/1 -> InertiaIdentification/3(g_b)

== system ACStesbed1/TestBedComputer/ModelCentralComputer/SPAttitude ==
  In1 : Inport
  Out1 : Outport
  wires:
  In1/1 -> Out1/1

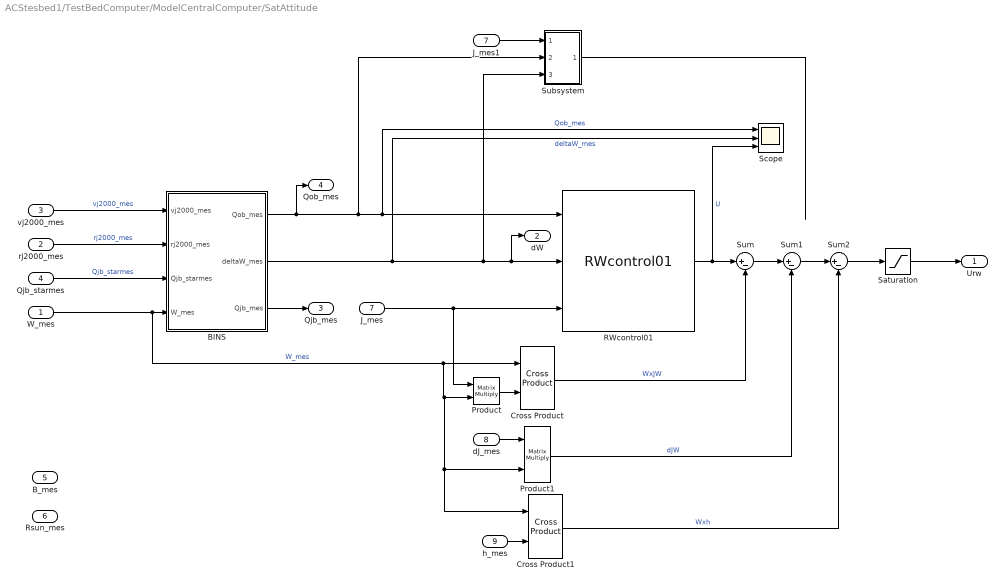
== system ACStesbed1/TestBedComputer/ModelCentralComputer/SatAttitude ==
  W_mes : Inport
  rj2000_mes : Inport  Port=2
  vj2000_mes : Inport  Port=3
  Qjb_starmes : Inport  Port=4
  B_mes : Inport  Port=5
  Rsun_mes : Inport  Port=6
  J_mes : Inport  Port=7
  dJ_mes : Inport  Port=8
  h_mes : Inport  Port=9
  BINS : Subsystem
  Cross Product : vrlib/Utilities/Cross Product
  Cross Product1 : vrlib/Utilities/Cross Product
  J_mes1 : InportShadow  Port=7
  Product : Product  Multiplication=Matrix(*)
  Product1 : Product  Multiplication=Matrix(*)
  RWcontrol01 : satellite_control_lib/RWcontrol01  Kq=params.K1acs  Kw=params.K2acs
  Saturation : Saturate
  Scope : Scope  NumInputPorts=3
      settings: ShowLegends=on  YMin=-0.1~-0.0012~-0.45  YMax=1~0.0004~0.2  SaveName=ScopeData7
  Subsystem : Subsystem
  Sum : Sum  Inputs=|+-
  Sum1 : Sum  Inputs=|+-
  Sum2 : Sum  Inputs=|+-
  Urw : Outport
  dW : Outport  Port=2
  Qjb_mes : Outport  Port=3
  Qob_mes : Outport  Port=4
  wires:
  RWcontrol01/1 -> Scope/3, Sum/1  "U"
  vj2000_mes/1 -> BINS/1(vj2000_mes)  "vj2000_mes"
  rj2000_mes/1 -> BINS/2(rj2000_mes)  "rj2000_mes"
  Qjb_starmes/1 -> BINS/3(Qjb_starmes)  "Qjb_starmes"
  W_mes/1 -> Cross Product1/1, Product1/2, Product/2, Cross Product/1, BINS/4(W_mes)  "W_mes"
  J_mes/1 -> Product/1, RWcontrol01/3
  BINS/1(Qob_mes) -> Qob_mes/1, Subsystem/2(In2), Scope/1, RWcontrol01/1  "Qob_mes"
  BINS/2(deltaW_mes) -> Scope/2, Subsystem/3(In3), dW/1, RWcontrol01/2  "deltaW_mes"
  J_mes1/1 -> Subsystem/1(In1)
  Subsystem/1(Out1) -> ?
  Saturation/1 -> Urw/1
  Product/1 -> Cross Product/2
  Cross Product/1 -> Sum/2  "WxJW"
  Product1/1 -> Sum1/2  "dJW"
  Cross Product1/1 -> Sum2/2  "Wxh"
  Sum/1 -> Sum1/1
  Sum1/1 -> Sum2/1
  Sum2/1 -> Saturation/1
  h_mes/1 -> Cross Product1/2
  dJ_mes/1 -> Product1/1
  BINS/3(Qjb_mes) -> Qjb_mes/1

== system ACStesbed1/TestBedComputer/ModelObject/Inertia ==
  deltaD : Inport
  Add : Sum  Inputs=+|+++
  Constant : Constant  Value=zeros(3,3)
  Constant1 : Constant  Value=params.J_b
  Constant2 : Constant  Value=params.be1
  Constant3 : Constant  Value=params.be2
  Constant4 : Constant  Value=params.be3
  Constant5 : Constant  Value=params.rho1
  Constant6 : Constant  Value=params.rho2
  Constant7 : Constant  Value=params.rho3
  Demux : Demux  Outputs=3
  deltaJ1 : Subsystem
  deltaJ2 : Subsystem
  deltaJ3 : Subsystem
  Inertia : Outport
  dInertia : Outport  Port=2
  wires:
  Constant/1 -> dInertia/1
  Constant1/1 -> Add/1  "J0"
  deltaD/1 -> Demux/1
  deltaJ1/1(deltaJ) -> Add/2  "deltaJ1"
  deltaJ2/1(deltaJ) -> Add/3  "deltaJ2"
  deltaJ3/1(deltaJ) -> Add/4  "deltaJ3"
  Add/1 -> Inertia/1  "J0+sum(deltaJ)"
  Demux/1 -> deltaJ1/1(d)
  Demux/2 -> deltaJ2/1(d)
  Demux/3 -> deltaJ3/1(d)
  Constant4/1 -> deltaJ3/2(e)
  Constant3/1 -> deltaJ2/2(e)
  Constant2/1 -> deltaJ1/2(e)
  Constant7/1 -> deltaJ3/3(rho)
  Constant6/1 -> deltaJ2/3(rho)
  Constant5/1 -> deltaJ1/3(rho)

== system ACStesbed1/TestBedComputer/ModelObject/OrbitalBasis ==
  vj2000 : Inport
  rj2000 : Inport  Port=2
  Cross Product : vrlib/Utilities/Cross Product
  Cross Product1 : vrlib/Utilities/Cross Product
  Direction Cosine Matrix to Quaternions : aerolibtransform2/Direction Cosine Matrix  to Quaternions
  Matrix Concatenate : Concatenate  NumInputs=3  Mode=Multidimensional array  ConcatenateDimension=2
  Normalize Vector : vrlib/Utilities/Normalize Vector  maxzero=0.00001
  Normalize Vector1 : vrlib/Utilities/Normalize Vector  maxzero=0.00001
  Quaternion Conjugate : aerolibutil/Quaternion Conjugate
  Qjo : Outport
  wires:
  Cross Product1/1 -> Matrix Concatenate/1  "iorb"
  Normalize Vector/1 -> Matrix Concatenate/2, Cross Product1/1  "jorb"
  Matrix Concatenate/1 -> Direction Cosine Matrix to Quaternions/1  "DCMjo"
  rj2000/1 -> Normalize Vector/1, Cross Product/2
  vj2000/1 -> Cross Product/1
  Direction Cosine Matrix to Quaternions/1 -> Quaternion Conjugate/1  "Qjo(in J frame)"
  Normalize Vector1/1 -> Matrix Concatenate/3, Cross Product1/2  "korb"
  Cross Product/1 -> Normalize Vector1/1
  Quaternion Conjugate/1 -> Qjo/1  "Qjo"

== system ACStesbed1/TestBedComputer/ModelObject/TestBedDynamics ==
  M : Inport
  Inertia : Inport  Port=2
  dInertia : Inport  Port=3
  Constant : Constant  Value=params.W_b
  Constant1 : Constant  Value=params.Qjb
  Cross Product : vrlib/Utilities/Cross Product
  Discrete-Time Integrator : DiscreteIntegrator  InitialConditionSource=external  ICPrevOutput=DiscIntNeverNeededParam  ICPrevScaledInput=DiscIntNeverNeededParam
  Divide : Product  Inputs=/*  Multiplication=Matrix(*)
  Inertia1 : InportShadow  Port=2
  Product : Product  Multiplication=Matrix(*)
  Product1 : Product  Multiplication=Matrix(*)
  Scope : Scope  NumInputPorts=2
      settings: ShowLegends=on  YMin=-0.0011~-0.01  YMax=0.0001~0.09  SaveName=ScopeData8
  Sum : Sum  Inputs=+--
  quatint : Subsystem
  Qjb : Outport
  Omega : Outport  Port=2
  wires:
  Sum/1 -> Divide/2
  Inertia1/1 -> Divide/1
  Divide/1 -> Discrete-Time Integrator/1  "dOmega"
  Constant/1 -> Discrete-Time Integrator/2
  Product/1 -> Sum/2  "dI*Omega"
  dInertia/1 -> Product/1
  Constant1/1 -> quatint/2(q_init)
  quatint/1(q) -> Qjb/1  "Qjb"
  Inertia/1 -> Product1/1
  Product1/1 -> Cross Product/2
  Cross Product/1 -> Sum/3  "Omega x I*Omega"
  Discrete-Time Integrator/1 -> Scope/1, quatint/1(p q r), Cross Product/1, Product/2, Product1/2, Omega/1  "W"
  M/1 -> Scope/2, Sum/1  "M"

== system ACStesbed1/TestBedComputer/ModelObject/Torques ==
  InData : Inport
  Add1 : Sum  Inputs=4
  Bus Selector : BusSelector  OutputSignals=signal2.signal1.dh,signal1.W,signal2.signal1.h,signal2.signal1.L
  ChangeMe1 : Constant  Value=[0 0 0]
  Saturation : Saturate  UpperLimit=1  LowerLimit=-1
  Tm : Subsystem
  Tothers : Subsystem
  Trw : Subsystem
  T : Outport
  wires:
  InData/1 -> Bus Selector/1
  Bus Selector/4 -> Tm/1(L)  "<L>"
  Add1/1 -> T/1
  Bus Selector/1 -> Trw/1(dh)  "<dh>"
  Bus Selector/2 -> Trw/2(W)  "<W>"
  Bus Selector/3 -> Trw/3(h)  "<h>"
  Trw/1(Trw) -> Saturation/1  "Trw_"
  Tm/1(Tm) -> ?  "Tm"
  Tothers/1(Tothers) -> ?  "Tothers"
  ChangeMe1/1 -> Tothers/1(Something), Tm/3(Ldisturb), Tm/2(B)
  Saturation/1 -> Add1/1

== system ACStesbed1/CentralComputer/SatAttitude/BINS/BINS correction ==
  Qjb_starmes : Inport
  Qjb_mes : Inport  Port=2
  Quaternion Conjugate : aerolibutil/Quaternion Conjugate
  Quaternion Conjugate1 : aerolibutil/Quaternion Conjugate
  Quaternion Multiplication : aerolibutil/Quaternion Multiplication
  Quaternion Multiplication1 : aerolibutil/Quaternion Multiplication
  Qjb_corrected : Outport
  wires:
  Quaternion Multiplication1/1 -> Qjb_corrected/1  "Qjb_corrected"
  Quaternion Conjugate1/1 -> Quaternion Multiplication1/1
  Qjb_mes/1 -> Quaternion Multiplication1/2, Quaternion Multiplication/2
  Quaternion Multiplication/1 -> Quaternion Conjugate1/1  "Nbb_mes"
  Qjb_starmes/1 -> Quaternion Conjugate/1
  Quaternion Conjugate/1 -> Quaternion Multiplication/1  "conjQjb_starmes"

== system ACStesbed1/CentralComputer/SatAttitude/BINS/Calc Qob ==
  Qjo : Inport
  Qjb : Inport  Port=2
  Quaternion Inverse : aerolibutil/Quaternion Inverse
  Quaternion Multiplication : aerolibutil/Quaternion Multiplication
  Qob : Outport
  wires:
  Qjb/1 -> Quaternion Multiplication/2  "Qjb"
  Qjo/1 -> Quaternion Inverse/1  "Qjo"
  Quaternion Inverse/1 -> Quaternion Multiplication/1
  Quaternion Multiplication/1 -> Qob/1
